simulink model "F16ASYM_Controlled_ACC"  (R2012b)
settings: Solver=ode3  SolverMode=SingleTasking  StartTime=0.0  StopTime=inf  FixedStep=T_sim  RelTol=1e-3
InitFcn:
  | load('NN_c_weights_Last_stable.mat')
values from neighbouring files (symbols this model uses):
  a1 = fitresult.p1    [Stall_protection.m]
  alpha_map_eval = ones(size(M_eval))*NaN    [Auto_trim_aid.m]    (also in Autotrim_maps.mat = [nan nan 0.277598136245 0.119432432992 0.0579479097061 0.027)
  beta_map_eval = ones(size(M_eval))*NaN    [Auto_trim_aid.m]    (also in Autotrim_maps.mat = [nan nan -0.00151549403324 0.00117807579006 -0.0052086799721)
  C_L_0 = fitresult.p2    [Stall_protection.m]
  G_eval = NaN*ones(size(M_sq,2),size(H_sq,2))    [Stall_protection.m]
  H_sq = unique(sort(H_sq))    [Stall_protection.m]
  H_sq_autotrim = min( F_envelope.H_1g):2000:max(F_envelope.H_1g)    [Auto_trim_aid.m]    (also in Autotrim_maps.mat = [0 2000 4000 6000 8000 10000 12000 14000 16000 18000])
  K_b_ACC = params(3)    [Cost_function.m]
  K_b_q = params(4)    [Cost_function.m]
  learning = 20    [Scheduling_desing.m]
  M_sq = unique(sort(M_sq))    [Stall_protection.m]
  M_sq_autotrim = 0:0.1:max(F_envelope.M_1g)    [Auto_trim_aid.m]    (also in Autotrim_maps.mat = [0 0.1 0.2 0.3 0.4 0.5 0.6 0.7 0.8 0.9 1 1.1 ... (21 element)
  Model_used_flag = 1    [Scheduling_desing.m]
  reg_param = 1    [Scheduling_desing.m]
  T_sim = 0.04    [Run_me.m]    (also in Scheduling_desing.m = 0.02)
  tau_ACC = params(1)    [Cost_function.m]
  tau_q = params(2)    [Cost_function.m]
  V_Comp_A_w_z_last = [-0.043311742939 0.0085685727899 -0.0213735657625 0.0330213821126 -0.0306555996667 -0.00573122365227 -0.0106441480787 0.0329440631876 0.0177121952361 -0.0290685435098 -0.0181457235686 -0.0361990502411 ... (1250 elements, 50x25)]    [NN_c_weights_Last_stable.mat]
  V_Comp_last = [-0.0421958473648 0.0184516098779 -0.0436695953504 -0.041154016657 0.00216882652165 -0.0388561228631 0.0327521861474 0.0326079628857 0.0227071838361 -0.0338588476214 0.0161615063846 0.00186003522421 ... (1250 elements, 50x25)]    [NN_c_weights_Last_stable.mat]
  velocity = M_eval(I,J)*a    [Auto_trim_aid.m]    (also in Scheduling_desing.m = M_eval_sche(I,J)*a)
  W_Comp_A_w_z_last = [-0.00689921461652 0.00234704735165 -0.000126421245896 0.00121944724496 6.17702028018e-05 -0.000422762754226 -0.000228913732743 -1.1618795843e-05 7.94007436465e-05 0.000588815786054 2.98617078429e-05 -0.00020420127191 ... (153 elements, 3x51)]    [NN_c_weights_Last_stable.mat]
  W_Comp_last = [-0.00864477030284 0.000183920433695 -0.000300268209456 0.00178165628538 -0.000144806488148 -0.000715209966 -0.000733452792184 5.9552378004e-05 0.000293789747621 0.00184648331608 -0.000150090451416 -0.000741280397229 ... (153 elements, 3x51)]    [NN_c_weights_Last_stable.mat]
undefined symbols (not defined in the file or in its folder): B, DiscIntNeverNeededParam, fi_flag_Simulink, k_B, m_B, sigbuilder_block, Stall_curve, Theta_1_roll_last, Theta_2_roll_last, Theta_3_roll_last, trim_control, trim_state, trim_throttle, V_long_lastA_w_z, V_long_lastAoA, V_roll_last, V_roll_lastMOD, V_yaw_last, W_long_lastA_w_z, W_long_lastAoA, W_roll_last, W_roll_lastMOD, W_yaw_last
libraries: Adaptive_FaultTolerantControl x43, F16_Actuator_Library x14, dspsigops x13, simulink x8, dsparch4 x6, simulink_extras x5, aerolibatmos2 x5, aerolibtransform2 x5, dspmtrx3 x3, qcatlib x2, dspvision x2, dspsnks4 x2
(part 6 of 10)

== system F16ASYM_Controlled_ACC/Primary Controller/P controller + adaptive Isolated NN/On-line (adaptive) multi-layer NNs SIMPL ==
  v_ad^ prev : Inport
  All_meas : Inport  Port=2
  NN variables : Inport  Port=3
  Bus Selector : BusSelector  OutputSignals=p_chanel_vars,Long chanel,beta_r_chanel
  Long Chanel : Subsystem  Variant=on  OverrideUsingVariant=Long HL NN A_w_z
  Long_learning rate : Constant  Value=19.7  SampleTime=T_sim
  Long_reg param : Constant  Value=0.9  SampleTime=T_sim
  Mux : Mux  Inputs=3
  Roll NN : Subsystem  Variant=on  OverrideUsingVariant=Roll 1HL NN
  Roll_learning rate : Constant  Value=80  SampleTime=T_sim
  Roll_reg param : Constant  Value=0.5  SampleTime=T_sim
  Selector : Selector  InputPortWidth=3  IndexOptions=Index vector (dialog)  Indices=1  OutputSizes=1
  Selector1 : Selector  InputPortWidth=3  IndexOptions=Index vector (dialog)  Indices=2  OutputSizes=1
  Selector2 : Selector  InputPortWidth=3  IndexOptions=Index vector (dialog)  Indices=3  OutputSizes=1
  Yaw Chanel : Subsystem  Variant=on  OverrideUsingVariant=Yaw HL NN
  Yaw_learning rate : Constant  Value=20.5  SampleTime=T_sim
  Yaw_reg param : Constant  SampleTime=T_sim
  v_ad^ prev1 : InportShadow
  v_ad^ prev2 : InportShadow
  v_ad^ : Outport
  wires:
  Long Chanel/1(v_ad_comp) -> Mux/2
  Yaw Chanel/1(v_ad_comp) -> Mux/3
  Bus Selector/3 -> Yaw Chanel/2(Yaw_chanel vars)  "<beta_r_chanel>"
  Selector2/1 -> Yaw Chanel/1(v_ad^ prev)
  v_ad^ prev2/1 -> Selector2/1
  Yaw_reg param/1 -> Yaw Chanel/5(Yaw reg param)
  Yaw_learning rate/1 -> Yaw Chanel/4(Yaw_learning rate)
  Bus Selector/2 -> Long Chanel/2(Long_chanel vars)  "<Long chanel>"
  v_ad^ prev1/1 -> Selector1/1
  Long_reg param/1 -> Long Chanel/5(Long reg param)
  Long_learning rate/1 -> Long Chanel/4(Long_learning rate)
  Selector1/1 -> Long Chanel/1(v_ad^ prev)
  Roll_reg param/1 -> Roll NN/5(Roll reg param)
  Roll_learning rate/1 -> Roll NN/4(Roll_learning rate)
  Selector/1 -> Roll NN/1(v_ad^ prev)
  v_ad^ prev/1 -> Selector/1
  Mux/1 -> v_ad^/1
  Roll NN/1(v_ad_comp) -> Mux/1
  All_meas/1 -> Roll NN/3(All_meas), Long Chanel/3(All_meas), Yaw Chanel/3(All_meas)
  Bus Selector/1 -> Roll NN/2(p_chanel vars)  "<p_chanel_vars>"
  NN variables/1 -> Bus Selector/1

== system F16ASYM_Controlled_ACC/Primary Controller/P controller + adaptive Isolated NN/Sigmoid  ==
  In : Inport
  Display : Display
  Fcn1 : Fcn  Commented=on  Expr=2.0 ./ (1.0 + exp(-u(4)*u(1:3)))-1
  MATLAB Function : MATLAB Function  TreatAsAtomicUnit=on
  a : Constant  Value=a
  Out : Outport
  wires:
  MATLAB Function/1(y) -> Display/1, Out/1
  In/1 -> MATLAB Function/1(u)
  a/1 -> MATLAB Function/2(a)

== system F16ASYM_Controlled_ACC/Primary Controller/PI Primary Controller/Body Rates Controller ==
  p_ref : Inport
  q_ref : Inport  Port=2
  r_ref : Inport  Port=3
  All_meas : Inport  Port=4
  All Anti-windup signals : Inport  Port=5
  Bus Creator : BusCreator  Inputs=3
  Bus Creator1 : BusCreator  Inputs=3
  Bus Creator2 : BusCreator  Inputs=3
  Bus Selector : BusSelector  OutputSignals=signal1.omega_b meas (rad/s)
  Display : Display
  Mux : Mux  Inputs=3
  Ref Model and PI Controller P : Adaptive_FaultTolerantControl/Ref Model and PI Controller  delta=0  tau=0.2  y_i=trim_state(10)  K_f=0.8  K_a=3  Con_way=pro  omega_n=4  xi=0.5  Z1=-30  K_b=10  f_i=0.2  f_c=1
  Ref Model and PI Controller q : Adaptive_FaultTolerantControl/Ref Model and PI Controller  delta=trim_state(11)  tau=0.15  y_i=0  K_f=0.8  K_a=3  Con_way=pro  omega_n=4  xi=0.5  Z1=-30  K_b=5  f_i=0.1  f_c=1
  Ref Model and PI Controller r : Adaptive_FaultTolerantControl/Ref Model and PI Controller  delta=trim_state(12)  tau=0.2  y_i=0  K_f=0.8  K_a=3  Con_way=pro  omega_n=4  xi=0.5  Z1=-30  K_b=10  f_i=0.2  f_c=1
  Selector : Selector  InputPortWidth=3  IndexOptions=Index vector (dialog)  Indices=1  OutputSizes=1
  Selector1 : Selector  InputPortWidth=3  IndexOptions=Index vector (dialog)  Indices=2  OutputSizes=1
  Selector2 : Selector  InputPortWidth=3  IndexOptions=Index vector (dialog)  Indices=3  OutputSizes=1
  Selector3 : Selector  InputPortWidth=3  IndexOptions=Index vector (dialog)  Indices=1  OutputSizes=1
  Selector4 : Selector  InputPortWidth=3  IndexOptions=Index vector (dialog)  Indices=2  OutputSizes=1
  Selector5 : Selector  InputPortWidth=3  IndexOptions=Index vector (dialog)  Indices=3  OutputSizes=1
  Sum : Sum  Inputs=|+-
  Sum1 : Sum  Inputs=|+-
  Sum2 : Sum  Inputs=|+-
  Terminator : Terminator
  Terminator1 : Terminator
  Terminator2 : Terminator
  Angular acc des (rad/s^2) : Outport
  wires:
  Bus Creator2/1 -> Terminator2/1
  Sum2/1 -> Bus Creator2/3  "r_err"
  Ref Model and PI Controller r/4 -> Sum2/2
  Ref Model and PI Controller r/3 -> Bus Creator2/2, Sum2/1  "r_sf"
  Ref Model and PI Controller r/2 -> Bus Creator2/1  "r_sf_dot"
  Bus Creator1/1 -> Terminator1/1
  Sum1/1 -> Bus Creator1/3  "q_err"
  Ref Model and PI Controller q/4 -> Sum1/2
  Ref Model and PI Controller q/3 -> Bus Creator1/2, Sum1/1  "q_sf"
  Ref Model and PI Controller q/2 -> Bus Creator1/1  "q_sf_dot"
  Bus Creator/1 -> Terminator/1
  Sum/1 -> Bus Creator/3  "p_err"
  Ref Model and PI Controller P/4 -> Sum/2
  Ref Model and PI Controller P/3 -> Bus Creator/2, Sum/1  "p_sf"
  Ref Model and PI Controller P/2 -> Bus Creator/1  "p_sf_dot"
  Selector3/1 -> Ref Model and PI Controller P/3
  Selector5/1 -> Ref Model and PI Controller r/3
  Selector4/1 -> Ref Model and PI Controller q/3, Display/1
  All Anti-windup signals/1 -> Selector3/1, Selector5/1, Selector4/1
  Ref Model and PI Controller r/1 -> Mux/3
  Ref Model and PI Controller q/1 -> Mux/2
  r_ref/1 -> Ref Model and PI Controller r/1
  Selector2/1 -> Ref Model and PI Controller r/2
  Selector1/1 -> Ref Model and PI Controller q/2
  q_ref/1 -> Ref Model and PI Controller q/1
  Mux/1 -> Angular acc des (rad/s^2)/1
  Ref Model and PI Controller P/1 -> Mux/1
  Selector/1 -> Ref Model and PI Controller P/2
  p_ref/1 -> Ref Model and PI Controller P/1
  Bus Selector/1 -> Selector/1, Selector1/1, Selector2/1  "<omega_b meas (rad/s)>"
  All_meas/1 -> Bus Selector/1

== system F16ASYM_Controlled_ACC/Primary Controller/PI Primary Controller/Lat_dir Dyn Inversion: beta_dot->r_c ==
  beta_dot_c : Inport
  All_meas : Inport  Port=2
  A_w_y : Selector  InputPortWidth=3  IndexOptions=Index vector (dialog)  Indices=2  OutputSizes=1
  Bus Selector : BusSelector  OutputSignals=signal1.AoA meas (rad),signal1.omega_b meas (rad/s),signal1.V_TAS (m/s),signal2.A_w_CG
  Divide1 : Product  Inputs=**
  Divide3 : Product  Inputs=**
  Divide4 : Product  Inputs=/*
  Divide5 : Product  Inputs=*/
  Selector : Selector  InputPortWidth=3  IndexOptions=Index vector (dialog)  Indices=1  OutputSizes=1
  Trigonometric Function : Trigonometry  Operator=cos
  Trigonometric Function3 : Trigonometry  Operator=tan
  "q_c " : Sum  Inputs=-++
  r_c : Outport
  wires:
  Selector/1 -> Divide1/2
  Trigonometric Function3/1 -> Divide1/1
  beta_dot_c/1 -> Divide5/1
  Divide5/1 -> "q_c "/1
  Trigonometric Function/1 -> Divide5/2, Divide3/1
  Bus Selector/3 -> Divide3/2  "<V_TAS (m/s)>"
  Divide4/1 -> "q_c "/3
  Bus Selector/4 -> A_w_y/1  "<A_w_CG>"
  All_meas/1 -> Bus Selector/1
  A_w_y/1 -> Divide4/2
  Divide3/1 -> Divide4/1
  Divide1/1 -> "q_c "/2
  Bus Selector/2 -> Selector/1  "<omega_b meas (rad/s)>"
  Bus Selector/1 -> Trigonometric Function3/1, Trigonometric Function/1  "<AoA meas (rad)>"
  "q_c "/1 -> r_c/1

== system F16ASYM_Controlled_ACC/Primary Controller/PI Primary Controller/Long Dyn Inversion: alpha_dot ->q ==
  alpha_dot_c : Inport
  All_meas : Inport  Port=2
  Completed : Subsystem
  Manual Switch : ManualSwitch
  Simplified : Subsystem
  q_c : Outport
  wires:
  Manual Switch/1 -> q_c/1
  Simplified/1(q_c) -> Manual Switch/2
  Completed/1(q_c) -> Manual Switch/1
  All_meas/1 -> Completed/2(All_meas), Simplified/2(All_meas)
  alpha_dot_c/1 -> Completed/1(alpha_dot_c), Simplified/1(alpha_dot_c)

== system F16ASYM_Controlled_ACC/Primary Controller/PI Primary Controller/Longitudinal Controller: AoA or A_w_z ==
  A_w_z des : Inport
  AoA des (rad) : Inport  Port=2
  Anti-windup A_w_z : Inport  Port=3
  Anti-windup AoA : Inport  Port=4
  All meas : Inport  Port=5
  Longitudinal controller in A_w_z : Subsystem  VariantObject=Controller of A_w_z
  Longitudinal controller in AoA : Subsystem  VariantObject=Controller of AoA
  alpha_dot_c : Outport

== system F16ASYM_Controlled_ACC/SI and FDI/SI and FDI: Realistic/FDI: Assumed? ==
  note: Add noise, uncertainty and delay here!!!
  note: RECONFIGURATION PARAMETERS
      |
      | 24. mass  Estimated mass
      | 25. S_current_L
      | 26. S_current_R
      | 27. S_fin_current
      | 28. x_cg
      | 29. Jy
      | 30. Jxz
      | 31. Jz
      | 32. Jx
      | 33. EFF_el_L
      | 34. EFF_el_R
      | 35. EFF_ail_L
      | 36. EFF_ail_R
      | 37. EFF_rud
      | 38. EFF_lef_L
      | 39. EFF_lef_R
      | 40. Delta_C_Lift_X
      | 41. Delta_C_Drag_X
      | 42. Delta_C_m_X
  Inexistent Reconfig bus : Inport
  All  meas : Inport  Port=2
  Bus Selector : BusSelector  OutputSignals=Reconfig signal,Blockades,Blockade now
  ONLY Effectiveness : Selector  InputPortWidth=19  IndexOptions=Index vector (dialog)  Indices=10:16  OutputSizes=1
  Terminator : Terminator
  Blockades at : Outport
  Blockades now : Outport  Port=2
  Effectiveness : Outport  Port=3
  wires:
  ONLY Effectiveness/1 -> Effectiveness/1
  Bus Selector/3 -> Blockades now/1  "<Blockade now>"
  Bus Selector/2 -> Blockades at/1  "<Blockades>"
  Bus Selector/1 -> ONLY Effectiveness/1  "<Reconfig signal>"
  Inexistent Reconfig bus/1 -> Bus Selector/1
  All  meas/1 -> Terminator/1

== system F16ASYM_Controlled_ACC/SI and FDI/SI and FDI: Realistic/SI ==
  note: Include here a logic that takes into account P so if the estimation is very bad do something
  note: Something to be done here!!!
  note: No estimation on this yet
  note: No estimation on this yet
  note: INPUTS
      | States:
      |
      | 1. Altitude
      | 2. TAS velocity
      | 3. alpha in rad
      | 4. beta in rads
      | 5. P
      | 6. Q
      | 7. R
      | 8. Throttle
      | 9. Elevator_L in deg
      | 10. Elevator_R in deg
      | 11. Aileron_L
      | 12. Aileron_R
      | 13. Rudder
      | 14. LEF_L
      | 15. LEF_R
      |
      | RECONFIGURATION PARAMETERS
      |
      | 16. mass  Estimated mass
      | 17. S_current_L
      | 18. S_current_R
      | 19. S_fin_current
      | 20. x_cg
      | 21. Jy
      | 22. Jxz
      | 23. Jz
      | 24. Jx
      | 25. EFF_el_L
      | 26. EFF_el_R
      | 27. EFF_ail_L
      | 28 EFF_ail_R
      | 29. EFF_rud
      | 30. EFF_lef_L
      | 31. EFF_lef_R
      | 32. Delta_C_Lift_X
      | 33. Delta_C_Drag_X
      | 34. Delta_C_m_X
  Control Eff : Inport
  All meas : Inport  Port=2
  Control comms : Inport  Port=3
  Add : Sum
  Band-Limited White Noise : simulink/Sources/Band-Limited White Noise  Cov=0.0000005  Ts=T_sim  seed=[23341]
  Base-line model parameters : Constant  Commented=on  Value=[9295.44,27.87/2,27.87/2,6.578,0.3,75673.6,1331.4,85552.1,12874.8]
  Bus Selector1 : BusSelector  OutputSignals=signal1.Alt meas (m),signal1.V_TAS (m/s),signal1.AoA meas (rad),signal1.SS meas (rad),signal1.omega_b meas (rad/s)
  Bus Selector2 : BusSelector  OutputSignals=signal1.omega_b meas (rad/s)
  Demux : Demux  Outputs=3
  Derivative : Derivative  CoefficientInTFapproximation=900
  Mass properties estimated : Constant  Value=[9295.44,0.3,75673.6,1331.4,85552.1,12874.8]
  Memory : Memory  X0=1*eye(3)
  Memory1 : Memory  X0=[27.87/2,27.87/2,6.578]
  Mux : Mux  Inputs=3
  Mux1 : Mux  Inputs=3
  NO-deviations from base-line model : Constant  Value=zeros(1,3)
  Scope : Scope
      settings: ShowLegends=on  YMin=1  YMax=15  SaveName=ScopeData23
  Scope1 : Scope
      settings: YMin=-2.75  YMax=3  SaveName=ScopeData24
  Surfaces UKF estimator : MATLAB Function  TreatAsAtomicUnit=on
  f(x)  Mom Coefficients due to the dynamics: Coefficients model with control inputs : MATLABFcn  Commented=on  MATLABFcn=Moms_Coeff_Reconf_estimator  OutputDimensions=3  OutputSignalType=real
  Est Mass props : Outport
  Est Surfs : Outport  Port=2
  Est Aero changes : Outport  Port=3
  wires:
  Mass properties estimated/1 -> Est Mass props/1
  All meas/1 -> Bus Selector1/1, Bus Selector2/1
  Control Eff/1 -> Surfaces UKF estimator/10(Ctrl_effectiveness)
  Control comms/1 -> Surfaces UKF estimator/9(Control_def)
  Bus Selector1/1 -> Surfaces UKF estimator/4(Alt)  "<Alt meas (m)>"
  Bus Selector1/2 -> Surfaces UKF estimator/5(TAS)  "<V_TAS (m/s)>"
  Bus Selector1/3 -> Surfaces UKF estimator/6(AoA)  "<AoA meas (rad)>"
  Bus Selector1/4 -> Surfaces UKF estimator/7(SS)  "<SS meas (rad)>"
  Bus Selector1/5 -> Surfaces UKF estimator/8(omega_b)  "<omega_b meas (rad/s)>"
  Surfaces UKF estimator/2(S_l) -> Mux/1
  Surfaces UKF estimator/3(S_r) -> Mux/2
  Surfaces UKF estimator/4(S_f) -> Mux/3
  Mux/1 -> Demux/1, Est Surfs/1, Memory1/1
  Surfaces UKF estimator/1(P_out) -> Memory/1
  NO-deviations from base-line model/1 -> Surfaces UKF estimator/11(Deltas_Aero), Est Aero changes/1
  Memory/1 -> Surfaces UKF estimator/1(P)
  Memory1/1 -> Surfaces UKF estimator/2(X_ant)
  Bus Selector2/1 -> Add/2  "<omega_b meas (rad/s)>"
  Derivative/1 -> Scope1/1, Surfaces UKF estimator/3(Meas)
  Band-Limited White Noise/1 -> Add/1
  Add/1 -> Derivative/1
  Demux/1 -> Mux1/1  "Left_wing"
  Demux/2 -> Mux1/2  "Right_wing"
  Demux/3 -> Mux1/3  "Fin"
  Mux1/1 -> Scope/1

== system F16ASYM_Controlled_ACC/Stall protection A_z and AoA/AoA and load factor map/If Action Subsystem ==
  Action Port : ActionPort
  From Multimedia File : dspvision/From Multimedia File  inputFilename=C:\Users\David\Documents\Estudios y formación academica\Cranfield\Thesis F16\Work\Solutions\7dof Development\Used Functions\Stall_warning.mp3  loop=on  numPlays=inf  outputStreams=Audio only  videoDataType=single  audioDataType=int16  inheritSampleTime=off  userDefinedSampleTime=T_sim  noAudioOutput=off  isIntensityVideo=off  fourcc=RGB  colorVideoFormat=Separate color signals  outputEOF=off  dataOrg=Column-major  audioFrameSize=1024  computeAudioFrameSize=off  outSamplingMode=Frame based
  To Audio Device : dspsnks4/To Audio Device  deviceName=Default  inheritSampleRate=on  sampleRate=44100  deviceDatatype=Determine from input data type  autoBufferSize=on  bufferSize=4096  queueDuration=1.0
  wires:
  From Multimedia File/1 -> To Audio Device/1

== system F16ASYM_Controlled_ACC/Stall protection A_z and AoA/Using AoA/Prediction ==
  V_TAS : Inport
  Add : Sum
  Derivative : Derivative  CoefficientInTFapproximation=20
  T_pred : Gain  Gain=T_pred
  V_tas pred : Outport
  wires:
  V_TAS/1 -> Add/1, Derivative/1
  Derivative/1 -> T_pred/1
  T_pred/1 -> Add/2
  Add/1 -> V_tas pred/1

== system F16ASYM_Controlled_ACC/Stall protection A_z and AoA/Using AoA/Speed stall logic ==
  stall signal : Inport
  Clock : Clock
  Constant : Constant  Value=-0.5/5  SampleTime=-1
  Constant1 : Constant  Value=0
  Discrete-Time Integrator : DiscreteIntegrator  ExternalReset=rising  InitialCondition=1  SampleTime=T_sim  LimitOutput=on  UpperSaturationLimit=1  LowerSaturationLimit=0  ICPrevOutput=DiscIntNeverNeededParam  ICPrevScaledInput=DiscIntNeverNeededParam
  pusher : Switch  Threshold=11
  timered signal : Outport
  wires:
  stall signal/1 -> Discrete-Time Integrator/2
  Constant/1 -> Discrete-Time Integrator/1
  Discrete-Time Integrator/1 -> pusher/1
  pusher/1 -> timered signal/1
  Clock/1 -> pusher/2
  Constant1/1 -> pusher/3

== system F16ASYM_Controlled_ACC/Stall protection A_z and AoA/Using AoA/play stall warning ==
  Action Port : ActionPort  InitializeStates=reset  ActionType=then
  From Multimedia File : dspvision/From Multimedia File  inputFilename=C:\Users\David\Documents\Estudios y formación academica\Cranfield\Thesis F16\Work\Solutions\7dof Development\Used Functions\Stall_warning.mp3  loop=on  numPlays=inf  outputStreams=Audio only  videoDataType=single  audioDataType=int16  inheritSampleTime=off  userDefinedSampleTime=T_sim  noAudioOutput=off  isIntensityVideo=off  fourcc=RGB  colorVideoFormat=Separate color signals  outputEOF=off  dataOrg=Column-major  audioFrameSize=1024  computeAudioFrameSize=off  outSamplingMode=Frame based
  To Audio Device : dspsnks4/To Audio Device  deviceName=Default  inheritSampleRate=on  sampleRate=44100  deviceDatatype=Determine from input data type  autoBufferSize=on  bufferSize=4096  queueDuration=1.0
  wires:
  From Multimedia File/1 -> To Audio Device/1

== system F16ASYM_Controlled_ACC/Control allocator/Control allocator: NO RECONF/Leading Edge Flap:Symetric deflection/Creating    qbar // ps ==
  alt : Inport
  V : Inport  Port=2
  ISA Atmosphere Model : aerolibatmos2/ISA Atmosphere Model  custom=off  g=9.80665  gamma=1.4  R=287.0531  L=0.0065  h_trop=11000  h_strat=20000  rho0=1.225  P0=101325  T0=288.15
  Math Function1 : Math  Operator=square  SaturateOnIntegerOverflow=on
  Product : Product  Inputs=/*  SaturateOnIntegerOverflow=on  InputSameDT=on  OutDataTypeStr=Inherit: Same as first input
  Product5 : Product  Inputs=**  SaturateOnIntegerOverflow=on  InputSameDT=on  OutDataTypeStr=Inherit: Same as first input
  Terminator : Terminator
  Terminator1 : Terminator
  r2d4 : Gain  Gain=0.5  SaturateOnIntegerOverflow=on  OutDataTypeStr=Inherit: Same as input  ParamDataTypeStr=Inherit: Same as input
  qbar / ps : Outport
  wires:
  ISA Atmosphere Model/2 -> Terminator1/1
  ISA Atmosphere Model/1 -> Terminator/1
  ISA Atmosphere Model/3 -> Product/1
  ISA Atmosphere Model/4 -> Product5/1
  Product/1 -> qbar / ps/1
  V/1 -> Math Function1/1
  Product5/1 -> Product/2  "qbar"
  r2d4/1 -> Product5/2
  Math Function1/1 -> r2d4/1
  alt/1 -> ISA Atmosphere Model/1

== system F16ASYM_Controlled_ACC/Control allocator/Control allocator: RECONFIG/Blockades logic: Limits injetor/Block AT INFERIOR LIMIT ==
  Limit : Inport
  Blockades : Inport  Port=2
  Demux : Demux  Outputs=7
  Mux2 : Mux  Inputs=7
  Selector : Selector  InputPortWidth=7  IndexOptions=Index vector (dialog)  Indices=1  OutputSizes=1
  Selector1 : Selector  InputPortWidth=7  IndexOptions=Index vector (dialog)  Indices=2  OutputSizes=1
  Selector2 : Selector  InputPortWidth=7  IndexOptions=Index vector (dialog)  Indices=3  OutputSizes=1
  Selector3 : Selector  InputPortWidth=7  IndexOptions=Index vector (dialog)  Indices=4  OutputSizes=1
  Selector4 : Selector  InputPortWidth=7  IndexOptions=Index vector (dialog)  Indices=5  OutputSizes=1
  Selector5 : Selector  InputPortWidth=7  IndexOptions=Index vector (dialog)  Indices=6  OutputSizes=1
  Selector6 : Selector  InputPortWidth=7  IndexOptions=Index vector (dialog)  Indices=7  OutputSizes=1
  Switch{,1..6} (7 alike) : Switch  Threshold=0.5
  isNaN{,1..6} (7 alike) : RelationalOperator  Operator=isNaN  OutDataTypeStr=boolean
  Reconfig limits : Outport
  wires:
  [Blockades] -> Selector/1
  isNaN/1 -> Switch/2
  Demux/1 -> Switch/1
  Selector/1 -> Switch/3, isNaN/1
  [Blockades] -> Selector1/1
  isNaN1/1 -> Switch1/2
  Demux/2 -> Switch1/1
  Selector1/1 -> Switch1/3, isNaN1/1
  [Blockades] -> Selector2/1
  isNaN2/1 -> Switch2/2
  Demux/3 -> Switch2/1
  Selector2/1 -> Switch2/3, isNaN2/1
  [Blockades] -> Selector3/1
  isNaN3/1 -> Switch3/2
  Demux/4 -> Switch3/1
  Selector3/1 -> Switch3/3, isNaN3/1
  [Blockades] -> Selector4/1
  isNaN4/1 -> Switch4/2
  Demux/5 -> Switch4/1
  Selector4/1 -> Switch4/3, isNaN4/1
  [Blockades] -> Selector5/1
  isNaN5/1 -> Switch5/2
  Demux/6 -> Switch5/1
  Selector5/1 -> Switch5/3, isNaN5/1
  [Blockades] -> Selector6/1
  isNaN6/1 -> Switch6/2
  Demux/7 -> Switch6/1
  Selector6/1 -> Switch6/3, isNaN6/1
  Limit/1 -> Demux/1
  Mux2/1 -> Reconfig limits/1
  Blockades/1 -> [Blockades]
  Switch/1 -> Mux2/1  "Elevator_L"
  Switch1/1 -> Mux2/2
  Switch2/1 -> Mux2/3  "Aileron_L"
  Switch3/1 -> Mux2/4  "Aileron_R"
  Switch4/1 -> Mux2/5  "Rudder"
  Switch5/1 -> Mux2/6  "LEF_L"
  Switch6/1 -> Mux2/7

== system F16ASYM_Controlled_ACC/Control allocator/Control allocator: RECONFIG/Blockades logic: Limits injetor/Block AT SUPERIOR LIMIT ==
  Limit : Inport
  Blockades : Inport  Port=2
  Demux : Demux  Outputs=7
  Mux2 : Mux  Inputs=7
  Selector : Selector  InputPortWidth=7  IndexOptions=Index vector (dialog)  Indices=1  OutputSizes=1
  Selector1 : Selector  InputPortWidth=7  IndexOptions=Index vector (dialog)  Indices=2  OutputSizes=1
  Selector2 : Selector  InputPortWidth=7  IndexOptions=Index vector (dialog)  Indices=3  OutputSizes=1
  Selector3 : Selector  InputPortWidth=7  IndexOptions=Index vector (dialog)  Indices=4  OutputSizes=1
  Selector4 : Selector  InputPortWidth=7  IndexOptions=Index vector (dialog)  Indices=5  OutputSizes=1
  Selector5 : Selector  InputPortWidth=7  IndexOptions=Index vector (dialog)  Indices=6  OutputSizes=1
  Selector6 : Selector  InputPortWidth=7  IndexOptions=Index vector (dialog)  Indices=7  OutputSizes=1
  Switch{,1..6} (7 alike) : Switch  Threshold=0.5
  isNaN{,1..6} (7 alike) : RelationalOperator  Operator=isNaN  OutDataTypeStr=boolean
  Reconfig limits : Outport
  wires:
  Switch6/1 -> Mux2/7
  Switch5/1 -> Mux2/6  "LEF_L"
  Switch4/1 -> Mux2/5  "Rudder"
  Switch3/1 -> Mux2/4  "Aileron_R"
  Switch2/1 -> Mux2/3  "Aileron_L"
  Switch1/1 -> Mux2/2
  Switch/1 -> Mux2/1  "Elevator_L"
  Blockades/1 -> [Blockades]
  Mux2/1 -> Reconfig limits/1
  Limit/1 -> Demux/1
  Selector6/1 -> isNaN6/1, Switch6/3
  Demux/7 -> Switch6/1
  isNaN6/1 -> Switch6/2
  [Blockades] -> Selector6/1
  Selector5/1 -> isNaN5/1, Switch5/3
  Demux/6 -> Switch5/1
  isNaN5/1 -> Switch5/2
  [Blockades] -> Selector5/1
  Selector4/1 -> isNaN4/1, Switch4/3
  Demux/5 -> Switch4/1
  isNaN4/1 -> Switch4/2
  [Blockades] -> Selector4/1
  Selector3/1 -> isNaN3/1, Switch3/3
  Demux/4 -> Switch3/1
  isNaN3/1 -> Switch3/2
  [Blockades] -> Selector3/1
  Selector2/1 -> isNaN2/1, Switch2/3
  Demux/3 -> Switch2/1
  isNaN2/1 -> Switch2/2
  [Blockades] -> Selector2/1
  Selector1/1 -> isNaN1/1, Switch1/3
  Demux/2 -> Switch1/1
  isNaN1/1 -> Switch1/2
  [Blockades] -> Selector1/1
  Selector/1 -> isNaN/1, Switch/3
  Demux/1 -> Switch/1
  isNaN/1 -> Switch/2
  [Blockades] -> Selector/1

== system F16ASYM_Controlled_ACC/Control allocator/Control allocator: RECONFIG/Blockades logic: Limits injetor/Block NOW INFERIOR LIMIT ==
  Limit : Inport
  Blockade now : Inport  Port=2
  Last deflection (abs) : Inport  Port=3
  Demux : Demux  Outputs=7
  Mux2 : Mux  Inputs=7
  Selector1 : Selector  InputPortWidth=7  IndexOptions=Index vector (dialog)  Indices=1  OutputSizes=1
  Selector10 : Selector  InputPortWidth=7  IndexOptions=Index vector (dialog)  Indices=4  OutputSizes=1
  Selector11 : Selector  InputPortWidth=7  IndexOptions=Index vector (dialog)  Indices=5  OutputSizes=1
  Selector12 : Selector  InputPortWidth=7  IndexOptions=Index vector (dialog)  Indices=6  OutputSizes=1
  Selector13 : Selector  InputPortWidth=7  IndexOptions=Index vector (dialog)  Indices=7  OutputSizes=1
  Selector14 : Selector  InputPortWidth=7  IndexOptions=Index vector (dialog)  Indices=7  OutputSizes=1
  Selector2 : Selector  InputPortWidth=7  IndexOptions=Index vector (dialog)  Indices=2  OutputSizes=1
  Selector3 : Selector  InputPortWidth=7  IndexOptions=Index vector (dialog)  Indices=3  OutputSizes=1
  Selector4 : Selector  InputPortWidth=7  IndexOptions=Index vector (dialog)  Indices=4  OutputSizes=1
  Selector5 : Selector  InputPortWidth=7  IndexOptions=Index vector (dialog)  Indices=5  OutputSizes=1
  Selector6 : Selector  InputPortWidth=7  IndexOptions=Index vector (dialog)  Indices=6  OutputSizes=1
  Selector7 : Selector  InputPortWidth=7  IndexOptions=Index vector (dialog)  Indices=1  OutputSizes=1
  Selector8 : Selector  InputPortWidth=7  IndexOptions=Index vector (dialog)  Indices=2  OutputSizes=1
  Selector9 : Selector  InputPortWidth=7  IndexOptions=Index vector (dialog)  Indices=3  OutputSizes=1
  Switch{7..13} (7 alike) : Switch  Threshold=0.5
  Reconfig limits : Outport
  wires:
  Mux2/1 -> Reconfig limits/1
  Limit/1 -> Demux/1
  Selector13/1 -> Switch13/2
  [Blockade_now] -> Selector13/1
  Demux/7 -> Switch13/3
  Selector12/1 -> Switch12/2
  [Blockade_now] -> Selector12/1
  Demux/6 -> Switch12/3  "LEF_L"
  Selector11/1 -> Switch11/2
  [Blockade_now] -> Selector11/1
  Demux/5 -> Switch11/3  "Rudder"
  Selector10/1 -> Switch10/2
  [Blockade_now] -> Selector10/1
  Demux/4 -> Switch10/3  "Aileron_R"
  Selector9/1 -> Switch9/2
  [Blockade_now] -> Selector9/1
  Selector8/1 -> Switch8/2
  [Blockade_now] -> Selector8/1
  Demux/2 -> Switch8/3
  Selector7/1 -> Switch7/2
  [Blockade_now] -> Selector7/1
  Demux/1 -> Switch7/3  "Elevator_L"
  Blockade now/1 -> [Blockade_now]
  Last deflection (abs)/1 -> [Actual_defle]
  Demux/3 -> Switch9/3
  Switch7/1 -> Mux2/1
  Switch8/1 -> Mux2/2
  Switch9/1 -> Mux2/3
  Switch10/1 -> Mux2/4
  Switch11/1 -> Mux2/5
  Switch12/1 -> Mux2/6
  Switch13/1 -> Mux2/7
  [Actual_defle] -> Selector1/1
  Selector1/1 -> Switch7/1
  [Actual_defle] -> Selector2/1
  Selector2/1 -> Switch8/1
  Selector3/1 -> Switch9/1
  [Actual_defle] -> Selector3/1
  Selector4/1 -> Switch10/1
  [Actual_defle] -> Selector4/1
  Selector5/1 -> Switch11/1
  [Actual_defle] -> Selector5/1
  Selector6/1 -> Switch12/1
  [Actual_defle] -> Selector6/1
  Selector14/1 -> Switch13/1
  [Actual_defle] -> Selector14/1

== system F16ASYM_Controlled_ACC/Control allocator/Control allocator: RECONFIG/Blockades logic: Limits injetor/Block NOW SUPERIOR LIMIT ==
  Limit : Inport
  Blockade now : Inport  Port=2
  Last deflection (abs) : Inport  Port=3
  Demux : Demux  Outputs=7
  Mux2 : Mux  Inputs=7
  Selector1 : Selector  InputPortWidth=7  IndexOptions=Index vector (dialog)  Indices=1  OutputSizes=1
  Selector10 : Selector  InputPortWidth=7  IndexOptions=Index vector (dialog)  Indices=4  OutputSizes=1
  Selector11 : Selector  InputPortWidth=7  IndexOptions=Index vector (dialog)  Indices=5  OutputSizes=1
  Selector12 : Selector  InputPortWidth=7  IndexOptions=Index vector (dialog)  Indices=6  OutputSizes=1
  Selector13 : Selector  InputPortWidth=7  IndexOptions=Index vector (dialog)  Indices=7  OutputSizes=1
  Selector14 : Selector  InputPortWidth=7  IndexOptions=Index vector (dialog)  Indices=7  OutputSizes=1
  Selector2 : Selector  InputPortWidth=7  IndexOptions=Index vector (dialog)  Indices=2  OutputSizes=1
  Selector3 : Selector  InputPortWidth=7  IndexOptions=Index vector (dialog)  Indices=3  OutputSizes=1
  Selector4 : Selector  InputPortWidth=7  IndexOptions=Index vector (dialog)  Indices=4  OutputSizes=1
  Selector5 : Selector  InputPortWidth=7  IndexOptions=Index vector (dialog)  Indices=5  OutputSizes=1
  Selector6 : Selector  InputPortWidth=7  IndexOptions=Index vector (dialog)  Indices=6  OutputSizes=1
  Selector7 : Selector  InputPortWidth=7  IndexOptions=Index vector (dialog)  Indices=1  OutputSizes=1
  Selector8 : Selector  InputPortWidth=7  IndexOptions=Index vector (dialog)  Indices=2  OutputSizes=1
  Selector9 : Selector  InputPortWidth=7  IndexOptions=Index vector (dialog)  Indices=3  OutputSizes=1
  Switch{7..13} (7 alike) : Switch  Threshold=0.5
  Reconfig limits : Outport
  wires:
  [Actual_defle] -> Selector14/1
  Selector14/1 -> Switch13/1
  [Actual_defle] -> Selector6/1
  Selector6/1 -> Switch12/1
  [Actual_defle] -> Selector5/1
  Selector5/1 -> Switch11/1
  [Actual_defle] -> Selector4/1
  Selector4/1 -> Switch10/1
  [Actual_defle] -> Selector3/1
  Selector3/1 -> Switch9/1
  Selector2/1 -> Switch8/1
  [Actual_defle] -> Selector2/1
  Selector1/1 -> Switch7/1
  [Actual_defle] -> Selector1/1
  Switch13/1 -> Mux2/7
  Switch12/1 -> Mux2/6
  Switch11/1 -> Mux2/5
  Switch10/1 -> Mux2/4
  Switch9/1 -> Mux2/3
  Switch8/1 -> Mux2/2
  Switch7/1 -> Mux2/1
  Demux/3 -> Switch9/3
  Last deflection (abs)/1 -> [Actual_defle]
  Blockade now/1 -> [Blockade_now]
  Demux/1 -> Switch7/3  "Elevator_L"
  [Blockade_now] -> Selector7/1
  Selector7/1 -> Switch7/2
  Demux/2 -> Switch8/3
  [Blockade_now] -> Selector8/1
  Selector8/1 -> Switch8/2
  [Blockade_now] -> Selector9/1
  Selector9/1 -> Switch9/2
  Demux/4 -> Switch10/3  "Aileron_R"
  [Blockade_now] -> Selector10/1
  Selector10/1 -> Switch10/2
  Demux/5 -> Switch11/3  "Rudder"
  [Blockade_now] -> Selector11/1
  Selector11/1 -> Switch11/2
  Demux/6 -> Switch12/3  "LEF_L"
  [Blockade_now] -> Selector12/1
  Selector12/1 -> Switch12/2
  Demux/7 -> Switch13/3
  [Blockade_now] -> Selector13/1
  Selector13/1 -> Switch13/2
  Limit/1 -> Demux/1
  Mux2/1 -> Reconfig limits/1

== system F16ASYM_Controlled_ACC/Control allocator/Control allocator: RECONFIG/Leading Edge Flap:Symetric deflection/Creating    qbar // ps ==
  alt : Inport
  V : Inport  Port=2
  ISA Atmosphere Model : aerolibatmos2/ISA Atmosphere Model  custom=off  g=9.80665  gamma=1.4  R=287.0531  L=0.0065  h_trop=11000  h_strat=20000  rho0=1.225  P0=101325  T0=288.15
  Math Function1 : Math  Operator=square  SaturateOnIntegerOverflow=on
  Product : Product  Inputs=/*  SaturateOnIntegerOverflow=on  InputSameDT=on  OutDataTypeStr=Inherit: Same as first input
  Product5 : Product  Inputs=**  SaturateOnIntegerOverflow=on  InputSameDT=on  OutDataTypeStr=Inherit: Same as first input
  Terminator : Terminator
  Terminator1 : Terminator
  r2d4 : Gain  Gain=0.5  SaturateOnIntegerOverflow=on  OutDataTypeStr=Inherit: Same as input  ParamDataTypeStr=Inherit: Same as input
  qbar / ps : Outport
  wires:
  alt/1 -> ISA Atmosphere Model/1
  Math Function1/1 -> r2d4/1
  r2d4/1 -> Product5/2
  Product5/1 -> Product/2  "qbar"
  V/1 -> Math Function1/1
  Product/1 -> qbar / ps/1
  ISA Atmosphere Model/4 -> Product5/1
  ISA Atmosphere Model/3 -> Product/1
  ISA Atmosphere Model/1 -> Terminator/1
  ISA Atmosphere Model/2 -> Terminator1/1

== system F16ASYM_Controlled_ACC/F-16 Non-linear Plant/SYM and ASYM model: No reconfigurable/Leading Edge Flap:Symetric deflection/Creating    qbar // ps ==
  alt : Inport
  V : Inport  Port=2
  ISA Atmosphere Model : aerolibatmos2/ISA Atmosphere Model  custom=off  g=9.80665  gamma=1.4  R=287.0531  L=0.0065  h_trop=11000  h_strat=20000  rho0=1.225  P0=101325  T0=288.15
  Math Function1 : Math  Operator=square  SaturateOnIntegerOverflow=on
  Product : Product  Inputs=/*  SaturateOnIntegerOverflow=on  InputSameDT=on  OutDataTypeStr=Inherit: Same as first input
  Product5 : Product  Inputs=**  SaturateOnIntegerOverflow=on  InputSameDT=on  OutDataTypeStr=Inherit: Same as first input
  Terminator : Terminator
  Terminator1 : Terminator
  r2d4 : Gain  Gain=0.5  SaturateOnIntegerOverflow=on  OutDataTypeStr=Inherit: Same as input  ParamDataTypeStr=Inherit: Same as input
  qbar / ps : Outport
  wires:
  ISA Atmosphere Model/2 -> Terminator1/1
  ISA Atmosphere Model/1 -> Terminator/1
  ISA Atmosphere Model/3 -> Product/1
  ISA Atmosphere Model/4 -> Product5/1
  Product/1 -> qbar / ps/1
  V/1 -> Math Function1/1
  Product5/1 -> Product/2  "qbar"
  r2d4/1 -> Product5/2
  Math Function1/1 -> r2d4/1
  alt/1 -> ISA Atmosphere Model/1

== system F16ASYM_Controlled_ACC/F-16 Non-linear Plant/SYM and ASYM model: RECONFIGURABLE/Leading Edge Flap:Symetric deflection/Creating    qbar // ps ==
  alt : Inport
  V : Inport  Port=2
  ISA Atmosphere Model : aerolibatmos2/ISA Atmosphere Model  custom=off  g=9.80665  gamma=1.4  R=287.0531  L=0.0065  h_trop=11000  h_strat=20000  rho0=1.225  P0=101325  T0=288.15
  Math Function1 : Math  Operator=square  SaturateOnIntegerOverflow=on
  Product : Product  Inputs=/*  SaturateOnIntegerOverflow=on  InputSameDT=on  OutDataTypeStr=Inherit: Same as first input
  Product5 : Product  Inputs=**  SaturateOnIntegerOverflow=on  InputSameDT=on  OutDataTypeStr=Inherit: Same as first input
  Terminator : Terminator
  Terminator1 : Terminator
  r2d4 : Gain  Gain=0.5  SaturateOnIntegerOverflow=on  OutDataTypeStr=Inherit: Same as input  ParamDataTypeStr=Inherit: Same as input
  qbar / ps : Outport
  wires:
  alt/1 -> ISA Atmosphere Model/1
  Math Function1/1 -> r2d4/1
  r2d4/1 -> Product5/2
  Product5/1 -> Product/2  "qbar"
  V/1 -> Math Function1/1
  Product/1 -> qbar / ps/1
  ISA Atmosphere Model/4 -> Product5/1
  ISA Atmosphere Model/3 -> Product/1
  ISA Atmosphere Model/1 -> Terminator/1
  ISA Atmosphere Model/2 -> Terminator1/1

== system F16ASYM_Controlled_ACC/P controller + adaptive Crossed NN + AWU+Lim    in ACC /Body Rates Controller/Ref Model and P Controller q/Reference Model ==
  y_ref : Inport
  Add : Sum  Inputs=|+-
  Integrator : Integrator  InitialCondition=trim_state(11)
  K_ref : Gain  Gain=1/tau_q
  y_c_dot : Outport
  y_c : Outport  Port=2
  wires:
  y_ref/1 -> Add/1
  Add/1 -> K_ref/1
  K_ref/1 -> Integrator/1, y_c_dot/1
  Integrator/1 -> y_c/1, Add/2

== system F16ASYM_Controlled_ACC/P controller + adaptive Crossed NN + AWU+Lim    in ACC /Longitudinal controller in A_w_z/Ref Model and P Controller/Reference Model ==
  y_ref : Inport
  Add : Sum  Inputs=|+-
  Integrator : Integrator
  K_ref : Gain  Gain=1/tau_ACC
  y_c_dot : Outport
  y_c : Outport  Port=2
  wires:
  y_ref/1 -> Add/1
  Add/1 -> K_ref/1
  K_ref/1 -> Integrator/1, y_c_dot/1
  Integrator/1 -> y_c/1, Add/2

== matlab function F16ASYM_Controlled_ACC/NDI/NDI: NO RECONFIG/Pre-Inverter ==
  data: p_dot_comm input; L_comm output; q_dot_comm input; r_dot_comm input; M_comm output; N_comm output; omega_b input
function [L_comm,M_comm,N_comm] = Pre_inverter(p_dot_comm,q_dot_comm,r_dot_comm,omega_b)
Jy  = 75673.6;
Jxz = 1331.4; 
Jz  = 85552.1;  
Jx  = 12874.8;
h_E = 216.9;

Gamma = Jx * Jz - (Jxz  * Jxz);
C1 = ((Jy - Jz)  * Jz  - (Jxz * Jxz))/ Gamma;
C2 = ((Jx - Jy + Jz ) * Jxz ) / Gamma;
C3 = Jz / Gamma;
C4 = Jxz / Gamma;
C5 = (Jz - Jx) / Jy;
C6 = Jxz / Jy ;
C7 = 1 / Jy;
C8 = (Jx * (Jx - Jy ) + Jxz * Jxz) / Gamma;
C9 = Jx / Gamma;



L_comm = -( C4*r_dot_comm+(C2*C9-C4*C8)*omega_b(1)*omega_b(2)+(C2*C4+C1*C9)*omega_b(2)*omega_b(3)-C9*p_dot_comm )/(C3*C9-C4^2);

M_comm = (q_dot_comm-C5*omega_b(1)*omega_b(3)+C6*omega_b(1)^2-C6*omega_b(3)^2 +C7*h_E*omega_b(3))/C7;

N_comm = ( C3*r_dot_comm-C4*p_dot_comm+(C4*C1+C3*C2)*omega_b(2)*omega_b(3)+(C4*C2-C3*C8)*omega_b(1)*omega_b(2)+(C4^2-C3*C9)*h_E*omega_b(2) )/(C3*C9-C4^2);

== matlab function F16ASYM_Controlled_ACC/SI and FDI/SI and FDI: Realistic/SI/Surfaces UKF estimator ==
  data: P input; P_out output; X_ant input; Meas input; Alt input; S_l output; TAS input; AoA input; SS input; omega_b input; Control_def input; Ctrl_effectiveness input; Deltas_Aero input; S_r output; S_f output
function [P_out,S_l,S_r,S_f] = UKF_estimator(P,X_ant,Meas,Alt,TAS,AoA,SS,omega_b,Control_def,Ctrl_effectiveness,Deltas_Aero)
% Control_def includes Throttle
% Meas are angular accelerations

m = 9295.44;
x_cg = 0.3;
Jy=75673.6;
Jxz=1331.4;
Jz=85552.1;
Jx=12874.8;

Ang_accels = zeros(3,1);
coder.extrinsic('Ang_accels_Reconf_estimator');
coder.extrinsic('schol');
coder.extrinsic('chol');

% Ang_accels = Ang_accels_Reconf_estimator([Alt,TAS,AoA,SS,omega_b',Control_def',m,  X_ant'  ,x_cg,Jy,Jxz,Jz,Jx,Ctrl_effectiveness',Deltas_Aero']');
% Ang_accels
% C_l = Ang_accels(1)
% C_m = Ang_accels(2)
% C_n = Ang_accels(3)


% S_l = 27.87/2;
% S_r=S_l;
% S_f = 6.578;
% P_out = P;


%% Filter UKF
% Init parameters 
F = eye(3);
Q = 0.005*eye(3); % Noise in the process (in surfaces)
R = 20*eye(3);   % Noise in the measures of angular acceleration

% Prediction . IT is a simple linear prediction. There is not need to do it
% in any other way because the result is the SAME
    x_pred=F*X_ant;
    x_pred(1) = max(0,min(x_pred(1),27.87/2));
    x_pred(2) = max(0,min(x_pred(2),27.87/2));
    x_pred(3) = max(0,min(x_pred(3),6.578));

    P_pred = F * P * F' + Q;

% Uncested Update
    % Measurement equations.
%     Ang_accels_Reconf_estimator([Alt,TAS,AoA,SS,omega_b',Control_def',m,  X_ant'  ,x_cg,Jy,Jxz,Jz,Jx,Ctrl_effectiveness',Deltas_Aero']')

    % Weight params
    L=size(X_ant,1);
    alpha = 1;  beta = 0;   kappa = 3 - L; % Supposed as optimals
    % %                 alpha = 0.6;  beta = 1.3;   kappa = 0.9; % Optimized by me
    
    % Generate_weights
        W_s = zeros(2*L+1,1);
        W_c = zeros(2*L+1,1);
        lambda = alpha^2 * (L + kappa) - L;
        for j=1:2*L+1
            if j==1
                W_s(j) = lambda / (L + lambda);
                W_c(j) = lambda / (L + lambda) + (1 - alpha^2 + beta);
            else
                W_s(j) = 1 / (2 * (L + lambda));
                W_c(j) = W_s(j);
            end
        end
        
    % Sigma_points
            flag = 0;
            A = zeros(size(P));
            [A,flag] = chol(P);
            A = A';
            if flag>0
                A = schol(P);
            end
        X = [zeros(size(x_pred)) A -A];
        X = sqrt(L + lambda)*X + repmat(x_pred,1,size(X,2));

    % Propagation with measurement equation (Model in this case)
        gamma_z = zeros(3,size(X,2));
        gamma_z(:,1) = Ang_accels_Reconf_estimator([Alt,TAS,AoA,SS,omega_b',Control_def',m,  X(:,1)'  ,x_cg,Jy,Jxz,Jz,Jx,Ctrl_effectiveness',Deltas_Aero']');
        for i=2:size(X,2)
%             [Alt,TAS,alpha,beta,omega_b',Control_def',m,  X(:,1)'  ,x_cg,Jy,Jxz,Jz,Jx,Ctrl_effectiveness',Deltas_Aero']
            gamma_z(:,i) = Ang_accels_Reconf_estimator([Alt,TAS,AoA,SS,omega_b',Control_def',m,  X(:,i)'  ,x_cg,Jy,Jxz,Jz,Jx,Ctrl_effectiveness',Deltas_Aero']');
        end
        
    % Update
    Z = zeros(size(gamma_z,1),1);
    Pzz  = zeros(size(gamma_z,1),size(gamma_z,1));
    Pxz  = zeros(size(x_pred,1),size(gamma_z,1));
    for i=1:size(X,2)
        Z = Z + W_s(i) * gamma_z(:,i);
    end
    for i=1:size(X,2)
        Pzz = Pzz + W_c(i) * (gamma_z(:,i) - Z) * (gamma_z(:,i) - Z)';
        Pxz = Pxz + W_c(i) * (X(1:size(x_pred,1),i) - x_pred) * (gamma_z(:,i) - Z)';
    end

    Pzz = Pzz + R;
    K = Pxz / Pzz;
    x_estimate = x_pred + K * (Meas - Z);
    P_out = P_pred - K * Pzz * K';
%     x_estimate
    S_l = x_estimate(1);
    S_r = x_estimate(2);
    S_f = x_estimate(3);

== matlab function F16ASYM_Controlled_ACC/Primary Controller/P  + Crossed NN + AWU+Lim + hand-over/P controller + adaptive Crossed NN + AWU+Lim    in ACC /Physical limitation/Ang Accel ==
  data: L input; p_dot output; q_dot output; r_dot output; M input; N input; omega_b input
function [p_dot,q_dot,r_dot] = Ang_accel(L,M,N,omega_b)
Jy  = 75673.6;
Jxz = 1331.4; 
Jz  = 85552.1;  
Jx  = 12874.8;
h_E = 216.9;

denom = Jx*Jz - Jxz*Jxz;

% % C1 = ((Jy - Jz)  * Jz  - (Jxz * Jxz))/ Gamma;
% % C2 = ((Jx - Jy + Jz ) * Jxz ) / Gamma;
% % C3 = Jz / Gamma;
% % C4 = Jxz / Gamma;
% % C5 = (Jz - Jx) / Jy;
% % C6 = Jxz / Jy ;
% % C7 = 1 / Jy;
% % C8 = (Jx * (Jx - Jy ) + Jxz * Jxz) / Gamma;
% % C9 = Jx / Gamma;


p_dot =  (Jz*L + Jxz*N - (Jz*(Jz-Jy)+Jxz*Jxz)*omega_b(2)*omega_b(3) + Jxz*(Jx-Jy+Jz)*omega_b(1)*omega_b(2) + Jxz*omega_b(2)*h_E)/denom;

q_dot = (M + (Jz-Jx)*omega_b(1)*omega_b(3) - Jxz*(omega_b(1)*omega_b(1)-omega_b(3)*omega_b(3)) - omega_b(3)*h_E)/Jy;


r_dot = (Jx*N + Jxz*L + (Jx*(Jx-Jy)+Jxz*Jxz)*omega_b(1)*omega_b(2) - Jxz*(Jx-Jy+Jz)*omega_b(2)*omega_b(3) +  Jx*omega_b(2)*h_E)/denom;

== system F16ASYM_Controlled_ACC/Primary Controller/P  + Crossed NN + AWU+Lim + hand-over/P controller + adaptive Crossed NN + AWU+Lim    in ACC /Body Rates Controller ==
  p_ref : Inport
  q_ref : Inport  Port=2
  r_ref : Inport  Port=3
  All_meas : Inport  Port=4
  Bus Creator : BusCreator
  Bus Creator1 : BusCreator
  Bus Creator2 : BusCreator
  Bus Selector : BusSelector  OutputSignals=signal1.omega_b meas (rad/s)
  Display1 : Display
  Mux : Mux  Inputs=3
  Ref Model and P Controller p : Adaptive_FaultTolerantControl/Ref Model and P Controller  tau=0.1  y_i=trim_state(10)  K_f=1  K_b=7
  Ref Model and P Controller q : Adaptive_FaultTolerantControl/Ref Model and P Controller  tau=0.07  y_i=trim_state(11)  K_f=1  K_b=3
  Ref Model and P Controller r : Adaptive_FaultTolerantControl/Ref Model and P Controller  tau=0.2  y_i=trim_state(12)  K_f=1  K_b=4
  Selector : Selector  InputPortWidth=3  IndexOptions=Index vector (dialog)  Indices=1  OutputSizes=1
  Selector1 : Selector  InputPortWidth=3  IndexOptions=Index vector (dialog)  Indices=2  OutputSizes=1
  Selector2 : Selector  InputPortWidth=3  IndexOptions=Index vector (dialog)  Indices=3  OutputSizes=1
  Sum : Sum  Inputs=+-|
  Sum1 : Sum  Inputs=+-|
  Sum2 : Sum  Inputs=+-|
  q_chanel vars : Outport
  p_chanel vars : Outport  Port=2
  r_chanel vars : Outport  Port=3
  Angular acc des (rad/s^2) : Outport  Port=4
  wires:
  All_meas/1 -> Bus Selector/1
  Bus Selector/1 -> Selector/1, Selector1/1, Selector2/1  "<omega_b meas (rad/s)>"
  p_ref/1 -> Ref Model and P Controller p/1
  Selector/1 -> Ref Model and P Controller p/2
  Ref Model and P Controller p/1 -> Mux/1
  Mux/1 -> Angular acc des (rad/s^2)/1
  q_ref/1 -> Ref Model and P Controller q/1
  Selector1/1 -> Ref Model and P Controller q/2
  r_ref/1 -> Ref Model and P Controller r/1
  Ref Model and P Controller q/1 -> Mux/2
  Ref Model and P Controller r/1 -> Mux/3
  Ref Model and P Controller p/2 -> Bus Creator/1  "p_sf_dot"
  Ref Model and P Controller p/3 -> Sum/1, Bus Creator/2  "p_sf"
  Sum/1 -> Display1/1, Bus Creator/3  "p_err"
  Bus Creator/1 -> p_chanel vars/1
  Bus Creator1/1 -> q_chanel vars/1
  Bus Creator2/1 -> r_chanel vars/1
  Selector2/1 -> Ref Model and P Controller r/2
  Ref Model and P Controller p/4 -> Sum/2
  Ref Model and P Controller p/5 -> Bus Creator/4  "K_b_p"
  Ref Model and P Controller q/2 -> Bus Creator1/1  "q_sf_dot"
  Ref Model and P Controller q/3 -> Sum1/1, Bus Creator1/2  "q_sf"
  Sum1/1 -> Bus Creator1/3  "q_err"
  Ref Model and P Controller q/4 -> Sum1/2
  Ref Model and P Controller q/5 -> Bus Creator1/4  "K_b_q"
  Ref Model and P Controller r/2 -> Bus Creator2/1  "r_sf_dot"
  Ref Model and P Controller r/3 -> Sum2/1, Bus Creator2/2  "r_sf"
  Sum2/1 -> Bus Creator2/3  "r_err"
  Ref Model and P Controller r/4 -> Sum2/2
  Ref Model and P Controller r/5 -> Bus Creator2/4  "K_b_r"
